simulink library "pend_lib"  (Simulink 7.0)
values from neighbouring files (symbols this model uses):
  A = [0 1      0 0 ... (first row only)    [init_pend_ctrllin.m]
  b = [0 ... (first row only)    [init_pend_ctrllin.m]
  Vlqr = 1/(c(:,1)' * inv(eye(4) - ssPend_disc.A+ssPend_disc.b*klqr) * ssPend_disc.b + d(1,:))    [init_pend_ctrllin.m]
  x10 = 0    [init_pend_ctrllin.m]
  xlin0 = [x10; x20; x30; x40]    [init_pend_ctrllin.m]
undefined symbols (not defined in the file or in its folder): bur_block_callback_handler, dv, klqr, l, m, x0, x20, x30, x40
libraries: bur_blks x6, pend_lib x3, cstblocks x1
settings Model: Creator=Bernecker + Rainer Industrie Elektronik Ges.m.b.H.  ModifiedByFormat=Bernecker + Rainer Industrie Elektronik Ges.m.b.H.  LastModifiedBy=Bernecker + Rainer Industrie Elektronik Ges.m.b.H.

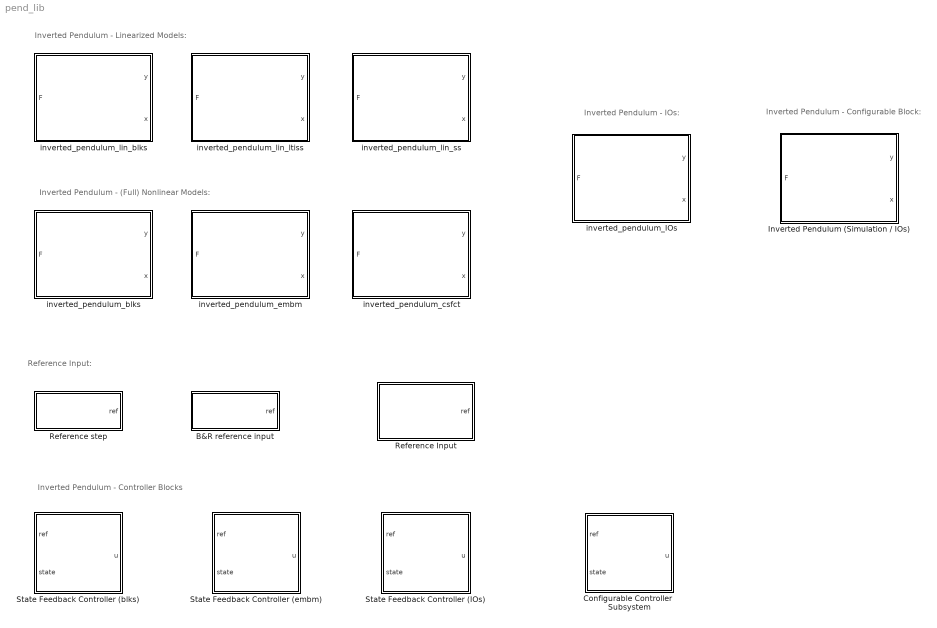
== system pend_lib ==
  note: Inverted Pendulum - Linearized Models:
  note: Inverted Pendulum - (Full) Nonlinear Models:
  note: Inverted Pendulum - Configurable Block:
  note: Inverted Pendulum - IOs:
  note: Reference Input:
  note: Inverted Pendulum - Controller Blocks
  B&R reference input : Subsystem
  Configurable Controller  Subsystem : Subsystem  BlockChoice=State Feedback Controller (blks)
      settings: TemplateBlock=self  MemberBlocks=State Feedback Controller (IOs),State Feedback Controller (blks),State Feedback Controller (embm)
  Inverted Pendulum (Simulation / IOs) : Subsystem  BlockChoice=inverted_pendulum_IOs
      settings: TemplateBlock=self  MemberBlocks=inverted_pendulum_IOs,inverted_pendulum_blks,inverted_pendulum_csfct,inverted_pendulum_embm,inverted_pendulum_lin_blks,inverted_pendulum_lin_ltiss,inverted_pendulum_lin_ss
      mask Display: image(imread('PEND.JPG'))
  Reference Input : Subsystem  BlockChoice=B&R reference input
      settings: TemplateBlock=self  MemberBlocks=B&R reference input,Reference step
  Reference step : Subsystem
  State Feedback Controller (IOs) : Subsystem
      mask Display: disp('Closed Loop\n Controller')
  State Feedback Controller (blks) : Subsystem
      mask Display: disp('Closed Loop\n Controller')
  State Feedback Controller (embm) : Subsystem
      mask Display: disp('Closed Loop\n Controller')
  inverted_pendulum_IOs : Subsystem  AncestorBlock=pend_lib/inverted_pendulum_lin_blks
      mask init:
      | % constants
      | g = 9.81;   % m/s^2 ... gravitational constant
      | 
      | % initializations
      | M = 100;   % kg ... mass of cart
      | m = 0.1;    % kg ... mass of pendulum (<< M)
      | l = 0.5;    % m  ... length of pendulum
      | 
      | % state variables & initial values
      | x1_0 = 0;   % m     ... position of cart
      | x2_0 = 0;   % m/s   ... speed of cart
      | x3_0 = 0;   % rad   ... angle of pendulum
      | x4_0 = 0;   % rad/s ... angular speed of pendulum
      | x_0 = [x1_0; x2_0; x3_0; x4_0];
      mask Display: image(imread('pend.jpg'))
  inverted_pendulum_blks : Subsystem
      mask init:
      | % constants
      | g = 9.81;   % m/s^2 ... gravitational constant
      | 
      | % initializations
      | M = 1000;   % kg ... mass of cart
      | m = 0.1;    % kg ... mass of pendulum (<< M)
      | l = 0.5;    % m  ... length of pendulum
      | 
      | % state variables & initial values
      | x1_0 = 0;   % m     ... position of cart
      | x2_0 = 0;   % m/s   ... speed of cart
      | x3_0 = 0;   % rad   ... angle of pendulum
      | x4_0 = 0;   % rad/s ... angular speed of pendulum
      | x_0 = [x1_0; x2_0; x3_0; x4_0];
      mask Display: image(imread('pend.jpg'))
  inverted_pendulum_csfct : Subsystem
      mask init: same as pend_lib/inverted_pendulum_blks
      mask Display: image(imread('PEND.JPG'))
  inverted_pendulum_embm : Subsystem
      mask init: same as pend_lib/inverted_pendulum_blks
      mask Display: image(imread('PEND.JPG'))
  inverted_pendulum_lin_blks : Subsystem
      mask init: same as pend_lib/inverted_pendulum_IOs
      mask Display: image(imread('pend.jpg'))
  inverted_pendulum_lin_ltiss : Subsystem
      mask init: same as pend_lib/inverted_pendulum_IOs
      mask Display: image(imread('pend.jpg'))
  inverted_pendulum_lin_ss : Subsystem
      mask init: same as pend_lib/inverted_pendulum_IOs
      mask Display: image(imread('pend.jpg'))

== system pend_lib/B&R reference input ==
  Input : bur_blks/Input  bur_var_name=ref  bur_var_description=Reference input  bur_scope=GLOBAL  bur_data_type=LREAL  bur_init_value=0  bur_init_value_bool=FALSE  bur_array_index=0  bur_old_var_name=ref  bur_var_memory=standard  bur_in_parameter=off
      settings: AttributesFormatString=_%<bur_scope> %<bur_data_type> %<bur_var_name>
  ref : Outport
  wires:
  Input/1 -> ref/1

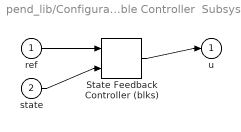
== system pend_lib/Configurable Controller  Subsystem ==
  ref : Inport
  state : Inport  Port=2
  State Feedback Controller (blks) : pend_lib/State Feedback Controller (blks)  SystemSampleTime=-1
  u : Outport
  wires:
  ref/1 -> State Feedback Controller (blks)/1
  state/1 -> State Feedback Controller (blks)/2
  State Feedback Controller (blks)/1 -> u/1

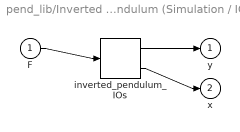
== system pend_lib/Inverted Pendulum (Simulation / IOs) ==
  F : Inport
  inverted_pendulum_IOs : pend_lib/inverted_pendulum_IOs  SystemSampleTime=-1
  y : Outport
  x : Outport  Port=2
  wires:
  F/1 -> inverted_pendulum_IOs/1
  inverted_pendulum_IOs/1 -> y/1
  inverted_pendulum_IOs/2 -> x/1

== system pend_lib/Reference Input ==
  B&R reference input : pend_lib/B&R reference input
  ref : Outport
  wires:
  B&R reference input/1 -> ref/1

== system pend_lib/Reference step ==
  Step : Step  Time=4  After=0.1  SampleTime=0
  ref : Outport
  wires:
  Step/1 -> ref/1

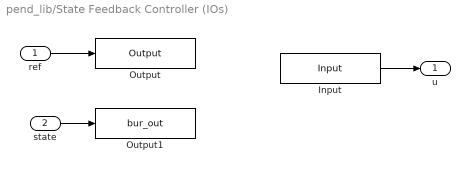
== system pend_lib/State Feedback Controller (IOs) ==
  ref : Inport
  state : Inport  Port=2
  Input : bur_blks/Input  bur_var_name=u_ctrl  bur_var_description=Controller manipulated variable  bur_scope=LOCAL  bur_data_type=LREAL  bur_init_value=0  bur_init_value_bool=FALSE  bur_array_index=0  bur_old_var_name=u_ctrl  bur_var_memory=standard  bur_in_parameter=off
      settings: AttributesFormatString=_%<bur_scope> %<bur_data_type> %<bur_var_name>
  Output : bur_blks/Output  bur_var_name=ref_ctrl  bur_var_description=Controller reference signal  bur_scope=LOCAL  bur_data_type=LREAL  bur_init_value=0  bur_init_value_bool=FALSE  bur_array_index=0  bur_old_var_name=ref_ctrl  bur_var_memory=standard
      settings: AttributesFormatString=_%<bur_scope> %<bur_data_type> %<bur_var_name>
  Output1 : S-Function  LoadFcn=bur_block_callback_handler('bur_block_output', 'bur_load');  FunctionName=bur_out  Parameters=bur_scope, bur_data_type, bur_init_value, bur_init_value_bool, bur_array_index, bur_var_name, bur_var_description  EnableBusSupport=off  mask(B&&R - Output Block){bur_var_name=state_ctrl, bur_var_description=Controller state feedback signal, bur_scope=LOCAL, bur_data_type=LREAL, bur_init_value=zeros(4,1), bur_init_value_bool=FALSE, bur_array_index=3, bur_old_var_name=state_ctrl}
      mask prompts: bur_var_name "Variable Name"; bur_var_description "Variable Description"; bur_scope "Variable Scope"; bur_data_type "Variable Data Type"; bur_init_value "Initial Value"; bur_init_value_bool "Initial Value"; bur_array_index "Array Dimension (0...Scalar)"; bur_old_var_name "Old Variable Name"
      mask help: Output interface for B&R Automation Studio process variable.
      mask init:
      | bur_block_callback_handler('bur_block_output', 'bur_confirm');
      settings: AttributesFormatString=_%<bur_scope> %<bur_data_type> %<bur_var_name>[0..%<bur_array_index>]  CopyFcn=bur_block_callback_handler('bur_block_output', 'bur_copy');
      mask Help: http://www.br-automation.com
      mask StyleString: edit,edit,popup(GLOBAL|LOCAL),popup(LREAL|REAL|SINT|USINT|INT|UINT|DINT|UDINT|BOOL),edit,popup(FALSE|TRUE),edit,edit
      mask CallbackString: bur_block_callback_handler('bur_block_output', 'bur_dialog_varname')|bur_block_callback_handler('bur_block_output', 'bur_dialog_vardescription')||bur_block_callback_handler('bur_block_output', 'bur_dialog_datatype')|bur_block_callback_handler('bur_block_output', 'bur_dialog_initvalue')||bur_block_callback_handler('bur_block_output', 'bur_dialog_arrayindex')|
      mask Display: color('orange'); disp('B&R OUT');
  u : Outport
  wires:
  ref/1 -> Output/1
  state/1 -> Output1/1
  Input/1 -> u/1

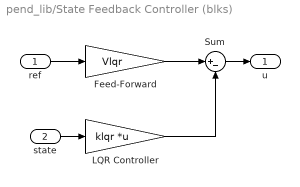
== system pend_lib/State Feedback Controller (blks) ==
  ref : Inport
  state : Inport  Port=2
  Feed-Forward : Gain  Gain=Vlqr
  LQR Controller : Gain  Gain=klqr  Multiplication=Matrix(K*u)
  Sum : Sum  Inputs=|+-
  u : Outport
  wires:
  state/1 -> LQR Controller/1
  Sum/1 -> u/1
  ref/1 -> Feed-Forward/1
  LQR Controller/1 -> Sum/2
  Feed-Forward/1 -> Sum/1

== system pend_lib/State Feedback Controller (embm) ==
  ref : Inport
  state : Inport  Port=2
  State Feedback Controller (embm) : Stateflow chart  TreatAsAtomicUnit=on
      settings: PermitHierarchicalResolution=ParametersOnly
  u : Outport
  wires:
  ref/1 -> State Feedback Controller (embm)/1(ref)
  state/1 -> State Feedback Controller (embm)/2(state)
  State Feedback Controller (embm)/1(u) -> u/1

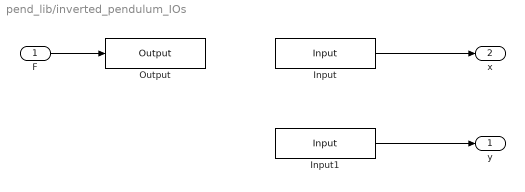
== system pend_lib/inverted_pendulum_IOs ==
  F : Inport
  Input : bur_blks/Input  bur_var_name=x  bur_var_description=Inverted pendulum state x  bur_scope=GLOBAL  bur_data_type=LREAL  bur_init_value=0  bur_init_value_bool=FALSE  bur_array_index=3  bur_old_var_name=x  bur_var_memory=standard  bur_in_parameter=off
      settings: AttributesFormatString=_%<bur_scope> %<bur_data_type> %<bur_var_name>[0..%<bur_array_index>]
  Input1 : bur_blks/Input  bur_var_name=y  bur_var_description=Inverted pendulum output y  bur_scope=GLOBAL  bur_data_type=LREAL  bur_init_value=0  bur_init_value_bool=FALSE  bur_array_index=1  bur_old_var_name=y  bur_var_memory=standard  bur_in_parameter=off
      settings: AttributesFormatString=_%<bur_scope> %<bur_data_type> %<bur_var_name>[0..%<bur_array_index>]
  Output : bur_blks/Output  bur_var_name=F  bur_var_description=Car force  bur_scope=GLOBAL  bur_data_type=LREAL  bur_init_value=0  bur_init_value_bool=FALSE  bur_array_index=0  bur_old_var_name=F  bur_var_memory=standard
      settings: AttributesFormatString=_%<bur_scope> %<bur_data_type> %<bur_var_name>
  y : Outport
  x : Outport  Port=2
  wires:
  F/1 -> Output/1
  Input/1 -> x/1
  Input1/1 -> y/1

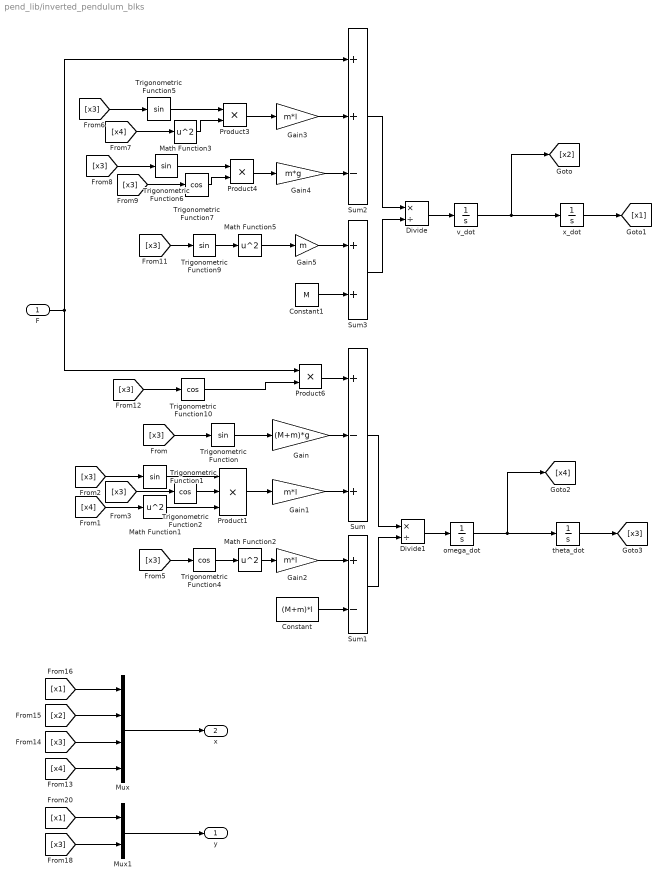
== system pend_lib/inverted_pendulum_blks ==
  F : Inport
  Constant : Constant  Value=(M+m)*l
  Constant1 : Constant  Value=M
  Divide : Product  Inputs=*/
  Divide1 : Product  Inputs=*/
  Gain : Gain  Gain=(M+m)*g
  Gain1 : Gain  Gain=m*l
  Gain2 : Gain  Gain=m*l
  Gain3 : Gain  Gain=m*l
  Gain4 : Gain  Gain=m*g
  Gain5 : Gain  Gain=m
  Math Function{1..3,5} (4 alike) : Math  Operator=square  SaturateOnIntegerOverflow=on
  Mux : Mux
  Mux1 : Mux  Inputs=2
  Product1 : Product  Inputs=3  RndMeth=Zero
  Product3 : Product  RndMeth=Zero
  Product4 : Product  RndMeth=Zero
  Product6 : Product  RndMeth=Zero
  Sum : Sum  Inputs=+-+
  Sum1 : Sum  Inputs=+-
  Sum2 : Sum  Inputs=++-
  Sum3 : Sum
  Trigonometric Function{,1,5..6,9} (5 alike) : Trigonometry
  Trigonometric Function{2,4,7,10} (4 alike) : Trigonometry  Operator=cos
  omega_dot : Integrator  InitialCondition=x0(4)
  theta_dot : Integrator  InitialCondition=x0(3)
  v_dot : Integrator  InitialCondition=x0(2)
  x_dot : Integrator  InitialCondition=x0(1)
  y : Outport
  x : Outport  Port=2
  wires:
  Sum2/1 -> Divide/1
  Sum3/1 -> Divide/2
  Sum1/1 -> Divide1/2
  Sum/1 -> Divide1/1
  Mux1/1 -> y/1
  [x3] -> Mux1/2
  [x1] -> Mux1/1
  [x4] -> Mux/4
  [x3] -> Mux/3
  [x2] -> Mux/2
  [x1] -> Mux/1
  Mux/1 -> x/1
  Math Function1/1 -> Product1/3
  [x4] -> Math Function1/1
  Trigonometric Function10/1 -> Product6/2
  [x3] -> Trigonometric Function10/1
  Product6/1 -> Sum/1
  Math Function5/1 -> Gain5/1
  Trigonometric Function9/1 -> Math Function5/1
  [x3] -> Trigonometric Function9/1
  Trigonometric Function7/1 -> Product4/2
  [x3] -> Trigonometric Function7/1
  Trigonometric Function6/1 -> Product4/1
  [x3] -> Trigonometric Function6/1
  [x4] -> Math Function3/1
  Math Function3/1 -> Product3/2
  Trigonometric Function5/1 -> Product3/1
  [x3] -> Trigonometric Function5/1
  theta_dot/1 -> [x3]
  Constant1/1 -> Sum3/2
  Gain5/1 -> Sum3/1
  Product4/1 -> Gain4/1
  Product3/1 -> Gain3/1
  Gain4/1 -> Sum2/3
  Gain3/1 -> Sum2/2
  Divide1/1 -> omega_dot/1
  omega_dot/1 -> theta_dot/1, [x4]
  Math Function2/1 -> Gain2/1
  Trigonometric Function4/1 -> Math Function2/1
  [x3] -> Trigonometric Function4/1
  Trigonometric Function2/1 -> Product1/2
  [x3] -> Trigonometric Function2/1
  Trigonometric Function1/1 -> Product1/1
  [x3] -> Trigonometric Function1/1
  Trigonometric Function/1 -> Gain/1
  [x3] -> Trigonometric Function/1
  x_dot/1 -> [x1]
  Constant/1 -> Sum1/2
  Gain2/1 -> Sum1/1
  Product1/1 -> Gain1/1
  Gain1/1 -> Sum/3
  Gain/1 -> Sum/2
  Divide/1 -> v_dot/1
  v_dot/1 -> [x2], x_dot/1
  F/1 -> Sum2/1, Product6/1

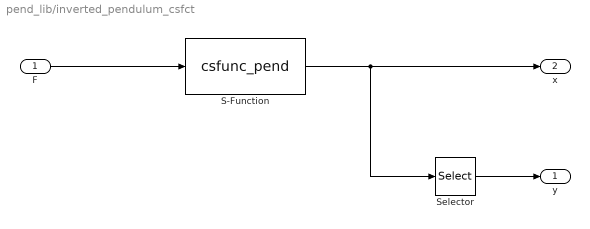
== system pend_lib/inverted_pendulum_csfct ==
  F : Inport
  S-Function : S-Function  FunctionName=csfunc_pend  Parameters=g, M, m, l, dv, x0  EnableBusSupport=off
  Selector : Selector  InputPortWidth=4  Indices=[1 3]
  y : Outport
  x : Outport  Port=2
  wires:
  F/1 -> S-Function/1
  S-Function/1 -> x/1, Selector/1
  Selector/1 -> y/1

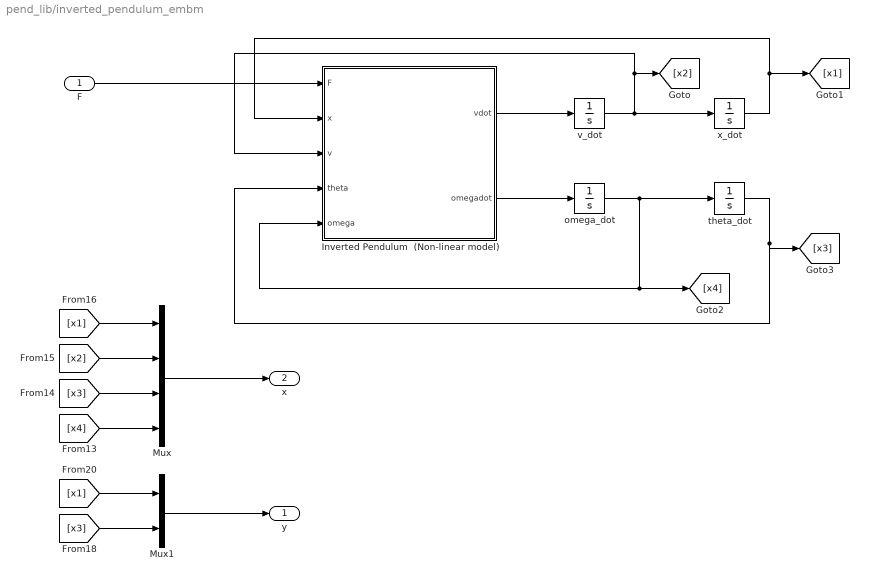
== system pend_lib/inverted_pendulum_embm ==
  F : Inport
  Inverted Pendulum  (Non-linear model) : Stateflow chart  TreatAsAtomicUnit=on
      settings: PermitHierarchicalResolution=ParametersOnly
  Mux : Mux
  Mux1 : Mux  Inputs=2
  omega_dot : Integrator  InitialCondition=x40
  theta_dot : Integrator  InitialCondition=x30
  v_dot : Integrator  InitialCondition=x20
  x_dot : Integrator  InitialCondition=x10
  y : Outport
  x : Outport  Port=2
  wires:
  theta_dot/1 -> [x3], Inverted Pendulum  (Non-linear model)/4(theta)
  Inverted Pendulum  (Non-linear model)/2(omegadot) -> omega_dot/1
  Inverted Pendulum  (Non-linear model)/1(vdot) -> v_dot/1
  F/1 -> Inverted Pendulum  (Non-linear model)/1(F)
  v_dot/1 -> [x2], Inverted Pendulum  (Non-linear model)/3(v), x_dot/1
  x_dot/1 -> [x1], Inverted Pendulum  (Non-linear model)/2(x)
  omega_dot/1 -> [x4], Inverted Pendulum  (Non-linear model)/5(omega), theta_dot/1
  Mux/1 -> x/1
  [x1] -> Mux/1
  [x2] -> Mux/2
  [x3] -> Mux/3
  [x4] -> Mux/4
  [x1] -> Mux1/1
  [x3] -> Mux1/2
  Mux1/1 -> y/1

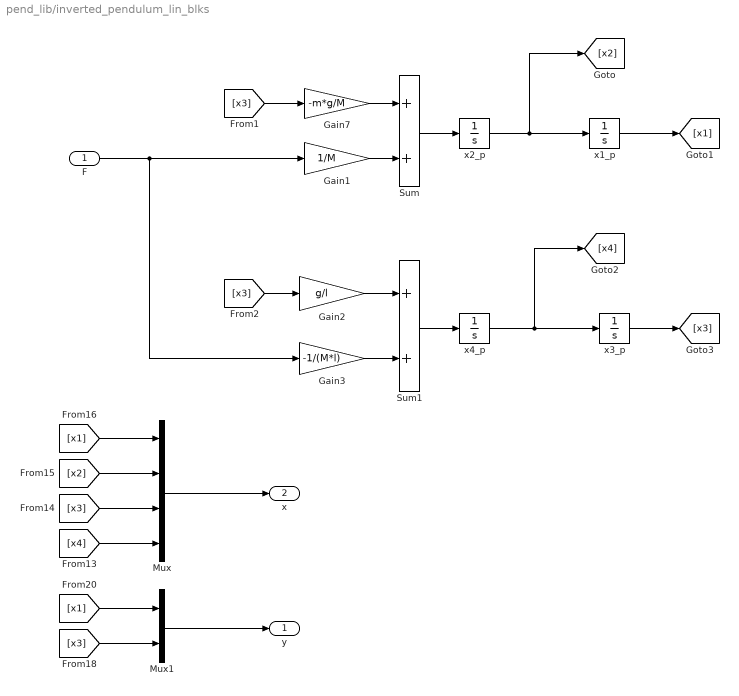
== system pend_lib/inverted_pendulum_lin_blks ==
  F : Inport
  Gain1 : Gain  Gain=1/M
  Gain2 : Gain  Gain=g/l
  Gain3 : Gain  Gain=-1/(M*l)
  Gain7 : Gain  Gain=-m*g/M
  Mux : Mux
  Mux1 : Mux  Inputs=2
  Sum : Sum
  Sum1 : Sum
  x1_p : Integrator  InitialCondition=xlin0(1)
  x2_p : Integrator  InitialCondition=xlin0(2)
  x3_p : Integrator  InitialCondition=xlin0(3)
  x4_p : Integrator  InitialCondition=xlin0(4)
  y : Outport
  x : Outport  Port=2
  wires:
  Mux1/1 -> y/1
  [x3] -> Mux1/2
  [x1] -> Mux1/1
  [x4] -> Mux/4
  [x3] -> Mux/3
  [x2] -> Mux/2
  [x1] -> Mux/1
  Mux/1 -> x/1
  x3_p/1 -> [x3]
  x4_p/1 -> x3_p/1, [x4]
  x1_p/1 -> [x1]
  x2_p/1 -> [x2], x1_p/1
  F/1 -> Gain1/1, Gain3/1
  [x3] -> Gain7/1
  Sum/1 -> x2_p/1
  Gain7/1 -> Sum/1
  Gain1/1 -> Sum/2
  Sum1/1 -> x4_p/1
  Gain2/1 -> Sum1/1
  [x3] -> Gain2/1
  Gain3/1 -> Sum1/2

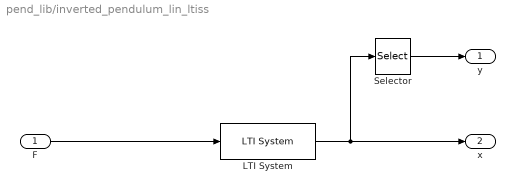
== system pend_lib/inverted_pendulum_lin_ltiss ==
  F : Inport
  LTI System : cstblocks/LTI System  sys=ssPend  IC=xlin0
  Selector : Selector  InputPortWidth=4  Indices=[1 3]
  y : Outport
  x : Outport  Port=2
  wires:
  F/1 -> LTI System/1
  LTI System/1 -> x/1, Selector/1
  Selector/1 -> y/1

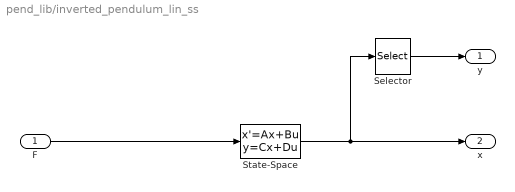
== system pend_lib/inverted_pendulum_lin_ss ==
  F : Inport
  Selector : Selector  InputPortWidth=4  Indices=[1 3]
  State-Space : StateSpace  A=A  B=b  C=eye(4)  D=zeros(4,1)  X0=xlin0
  y : Outport
  x : Outport  Port=2
  wires:
  Selector/1 -> y/1
  State-Space/1 -> Selector/1, x/1
  F/1 -> State-Space/1

== matlab function State Feedback Controller (embm)/State Feedback Controller (embm) ==
  data: ref input double; u output double; state input double; Vlqr parameter double; klqr parameter double
function u = fcn(ref, state, Vlqr, klqr)
%#eml

u = -klqr * state + Vlqr * ref;

== matlab function inverted_pendulum_embm/Inverted Pendulum (Non-linear model) ==
  data: F input double; vdot output double size=1; x input double; v input double; theta input double; omega input double; M parameter double; m parameter double; l parameter double; g parameter double; dv parameter double; omegadot output double size=1
function [vdot, omegadot] = fcn(F, x, v, theta, omega, M, m, l, g, dv)
%#eml

vdot = (-m*g*sin(theta)*cos(theta) + m*l*omega^2*sin(theta) + F) / (M+m*sin(theta)^2);
omegadot = ((M+m)*g*sin(theta) - (M+m)/(m*l)*dv*omega - cos(theta)*F - m*l*omega^2*sin(theta)*cos(theta)) / (M+m*sin(theta)^2)/l;
